simulink model "Position_Model"  (R2021a)
settings: Solver=VariableStepAuto  StartTime=0.0  StopTime=10.0  RelTol=1e-3
values from neighbouring files (symbols this model uses):
  Kr = 1.73    [TransferFunctionCode.m]    (also in run_steering_simulation.m)
  Kv = 0.53    [TransferFunctionCode.m]    (also in run_steering_simulation.m)
  phi_0 = 0    [run_steering_simulation.m]
  rhodot_d = 0.1    [run_steering_simulation.m]
  sigmar = 2.94    [TransferFunctionCode.m]    (also in run_steering_simulation.m)
  sigmav = 5.88    [TransferFunctionCode.m]    (also in run_steering_simulation.m)
  x_0 = 0    [run_steering_simulation.m]
  x_s = [0 3 6 10]    [run_steering_simulation.m]
  y_0 = 0    [run_steering_simulation.m]
  y_s = [0 0 3 3]    [run_steering_simulation.m]
libraries: pid_lib x3
settings Model: Creator=Brook Walls  LastModifiedBy=Brook Walls

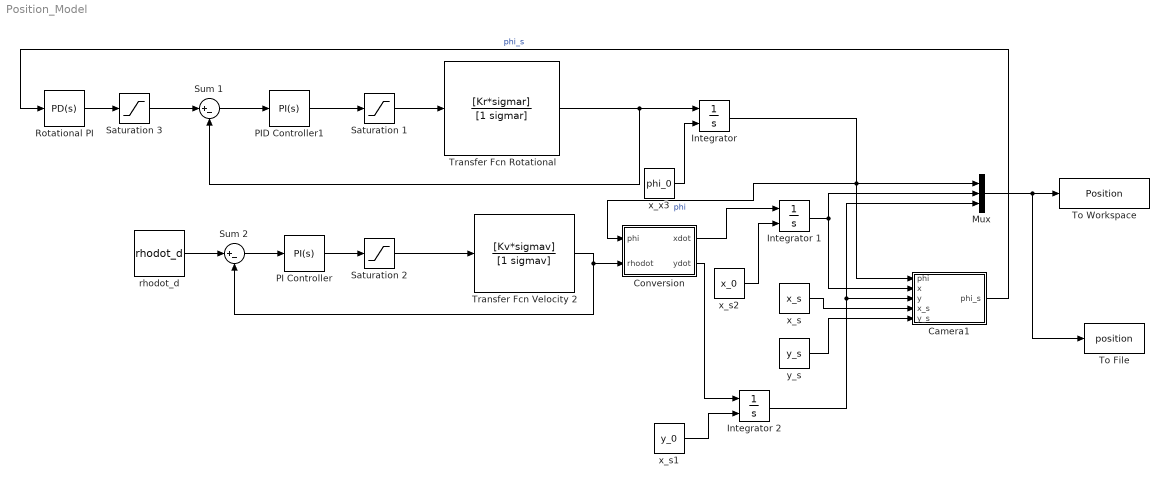
== system Position_Model ==
  Camera1 : MATLAB Function  TreatAsAtomicUnit=on  SystemSampleTime=.2
  Conversion : MATLAB Function  TreatAsAtomicUnit=on
  "Integrator " : Integrator  InitialConditionSource=external
  Integrator 1 : Integrator  InitialConditionSource=external
  Integrator 2 : Integrator  InitialConditionSource=external
  Mux : Mux  Inputs=3
  "PI Controller " : pid_lib/PID Controller  Controller=PI  Form=Parallel  TimeDomain=Continuous-time  UseExternalTs=off  SampleTime=-1  IntegratorMethod=Forward Euler  FilterMethod=Forward Euler  ControllerParametersSource=internal  P=3.69119211409962  I=0  D=0  UseFilter=on  N=100  TunerSelectOption=Transfer Function Based (PID Tuner App)  InitialConditionSource=internal  InitialConditionForIntegrator=0  InitialConditionForFilter=0  DifferentiatorICPrevScaledInput=0  ExternalReset=none  TrackingMode=off  Kt=1  LimitOutput=off  SatLimitsSource=internal  UpperSaturationLimit=inf  LowerSaturationLimit=-inf  LinearizeAsGain=on  AntiWindupMode=none  Kb=1  POutMin=[]  POutMax=[]  IOutMin=[]  IOutMax=[]  DOutMin=[]  DOutMax=[]  NOutMin=[]  NOutMax=[]  SumOutMin=[]  SumOutMax=[]  SaturationOutMin=[]  SaturationOutMax=[]  PParamMin=[]  PParamMax=[]  IParamMin=[]  IParamMax=[]  DParamMin=[]  DParamMax=[]  NParamMin=[]  NParamMax=[]  KbParamMin=[]  KbParamMax=[]  KtParamMin=[]  KtParamMax=[]  KbOutMin=[]  KbOutMax=[]  KtOutMin=[]  KtOutMax=[]  IntegratorOutMin=[]  IntegratorOutMax=[]  FilterOutMin=[]  FilterOutMax=[]  SumI1OutMin=[]  SumI1OutMax=[]  SumI2OutMin=[]  SumI2OutMax=[]  SumI3OutMin=[]  SumI3OutMax=[]  SumI4OutMin=[]  SumI4OutMax=[]  SumDOutMin=[]  SumDOutMax=[]  DifferentiatorOutMin=[]  DifferentiatorOutMax=[]  FilterDiffOutCoefMin=[]  FilterDiffOutCoefMax=[]  ReciprocalOutMin=[]  ReciprocalOutMax=[]  SumDenOutMin=[]  SumDenOutMax=[]  SumNumOutMin=[]  SumNumOutMax=[]  DivideOutMin=[]  DivideOutMax=[]  UdiffTsProdOutMin=[]  UdiffTsProdOutMax=[]  NTsProdOutMin=[]  NTsProdOutMax=[]  UintegralTsProdOutMin=[]  UintegralTsProdOutMax=[]  UngainTsProdOutMin=[]  UngainTsProdOutMax=[]  IntegratorContinuousStateAttributes=''  IntegratorStateMustResolveToSignalObject=off  IntegratorRTWStateStorageClass=Auto  FilterContinuousStateAttributes=''  FilterStateMustResolveToSignalObject=off  FilterRTWStateStorageClass=Auto  ParallelPVariant=InternalParameters  IdealPVariant=Disabled  IVariant=InternalParameters  DVariant=Disabled  IntegratorVariant=Continuous  SatVariant=Disabled  AWVariant=Passthrough  PCopyVariant=Disabled  TRVariant=Disabled  FdbkBlocksVariant=Forward  IdealPFdbkVariant=Disabled  SatFdbkVariant=Disabled  DerivativeFilterVariant=Disabled  NVariant=Disabled  NCopyVariant=Disabled_SignalSpec  FilterICVariant=Disabled  IntegratorICVariant=InternalICs  ExternalResetVariant=Disabled  TRSumVariant=Passthrough  SumFdbkVariant=Disabled  SumVariant=Sum_PI  TsampFilterVariant=InternalTs  TsampNgainVariant=Passthrough  TsampIntegralVariant=Passthrough  ExternalSaturationOutDataTypeStr=Inherit: Same as second input
  PID Controller1 : pid_lib/PID Controller  Controller=PI  Form=Parallel  TimeDomain=Continuous-time  UseExternalTs=off  SampleTime=-1  IntegratorMethod=Forward Euler  FilterMethod=Forward Euler  ControllerParametersSource=internal  P=2.17  I=0  D=0  UseFilter=on  N=100  TunerSelectOption=Transfer Function Based (PID Tuner App)  InitialConditionSource=internal  InitialConditionForIntegrator=0  InitialConditionForFilter=0  DifferentiatorICPrevScaledInput=0  ExternalReset=none  TrackingMode=off  Kt=1  LimitOutput=off  SatLimitsSource=internal  UpperSaturationLimit=inf  LowerSaturationLimit=-inf  LinearizeAsGain=on  AntiWindupMode=none  Kb=1  POutMin=[]  POutMax=[]  IOutMin=[]  IOutMax=[]  DOutMin=[]  DOutMax=[]  NOutMin=[]  NOutMax=[]  SumOutMin=[]  SumOutMax=[]  SaturationOutMin=[]  SaturationOutMax=[]  PParamMin=[]  PParamMax=[]  IParamMin=[]  IParamMax=[]  DParamMin=[]  DParamMax=[]  NParamMin=[]  NParamMax=[]  KbParamMin=[]  KbParamMax=[]  KtParamMin=[]  KtParamMax=[]  KbOutMin=[]  KbOutMax=[]  KtOutMin=[]  KtOutMax=[]  IntegratorOutMin=[]  IntegratorOutMax=[]  FilterOutMin=[]  FilterOutMax=[]  SumI1OutMin=[]  SumI1OutMax=[]  SumI2OutMin=[]  SumI2OutMax=[]  SumI3OutMin=[]  SumI3OutMax=[]  SumI4OutMin=[]  SumI4OutMax=[]  SumDOutMin=[]  SumDOutMax=[]  DifferentiatorOutMin=[]  DifferentiatorOutMax=[]  FilterDiffOutCoefMin=[]  FilterDiffOutCoefMax=[]  ReciprocalOutMin=[]  ReciprocalOutMax=[]  SumDenOutMin=[]  SumDenOutMax=[]  SumNumOutMin=[]  SumNumOutMax=[]  DivideOutMin=[]  DivideOutMax=[]  UdiffTsProdOutMin=[]  UdiffTsProdOutMax=[]  NTsProdOutMin=[]  NTsProdOutMax=[]  UintegralTsProdOutMin=[]  UintegralTsProdOutMax=[]  UngainTsProdOutMin=[]  UngainTsProdOutMax=[]  IntegratorContinuousStateAttributes=''  IntegratorStateMustResolveToSignalObject=off  IntegratorRTWStateStorageClass=Auto  FilterContinuousStateAttributes=''  FilterStateMustResolveToSignalObject=off  FilterRTWStateStorageClass=Auto  ParallelPVariant=InternalParameters  IdealPVariant=Disabled  IVariant=InternalParameters  DVariant=Disabled  IntegratorVariant=Continuous  SatVariant=Disabled  AWVariant=Passthrough  PCopyVariant=Disabled  TRVariant=Disabled  FdbkBlocksVariant=Forward  IdealPFdbkVariant=Disabled  SatFdbkVariant=Disabled  DerivativeFilterVariant=Disabled  NVariant=Disabled  NCopyVariant=Disabled_SignalSpec  FilterICVariant=Disabled  IntegratorICVariant=InternalICs  ExternalResetVariant=Disabled  TRSumVariant=Passthrough  SumFdbkVariant=Disabled  SumVariant=Sum_PI  TsampFilterVariant=InternalTs  TsampNgainVariant=Passthrough  TsampIntegralVariant=Passthrough  ExternalSaturationOutDataTypeStr=Inherit: Same as second input
  Rotational PI : pid_lib/PID Controller  Controller=PD  Form=Parallel  TimeDomain=Continuous-time  UseExternalTs=off  SampleTime=-1  IntegratorMethod=Forward Euler  FilterMethod=Forward Euler  ControllerParametersSource=internal  P=51.0923671487987  I=0  D=1.88750160017892  UseFilter=on  N=309.746780654974  TunerSelectOption=Transfer Function Based (PID Tuner App)  InitialConditionSource=internal  InitialConditionForIntegrator=0  InitialConditionForFilter=0  DifferentiatorICPrevScaledInput=0  ExternalReset=none  TrackingMode=off  Kt=1  LimitOutput=off  SatLimitsSource=internal  UpperSaturationLimit=inf  LowerSaturationLimit=-inf  LinearizeAsGain=on  AntiWindupMode=none  Kb=1  POutMin=[]  POutMax=[]  IOutMin=[]  IOutMax=[]  DOutMin=[]  DOutMax=[]  NOutMin=[]  NOutMax=[]  SumOutMin=[]  SumOutMax=[]  SaturationOutMin=[]  SaturationOutMax=[]  PParamMin=[]  PParamMax=[]  IParamMin=[]  IParamMax=[]  DParamMin=[]  DParamMax=[]  NParamMin=[]  NParamMax=[]  KbParamMin=[]  KbParamMax=[]  KtParamMin=[]  KtParamMax=[]  KbOutMin=[]  KbOutMax=[]  KtOutMin=[]  KtOutMax=[]  IntegratorOutMin=[]  IntegratorOutMax=[]  FilterOutMin=[]  FilterOutMax=[]  SumI1OutMin=[]  SumI1OutMax=[]  SumI2OutMin=[]  SumI2OutMax=[]  SumI3OutMin=[]  SumI3OutMax=[]  SumI4OutMin=[]  SumI4OutMax=[]  SumDOutMin=[]  SumDOutMax=[]  DifferentiatorOutMin=[]  DifferentiatorOutMax=[]  FilterDiffOutCoefMin=[]  FilterDiffOutCoefMax=[]  ReciprocalOutMin=[]  ReciprocalOutMax=[]  SumDenOutMin=[]  SumDenOutMax=[]  SumNumOutMin=[]  SumNumOutMax=[]  DivideOutMin=[]  DivideOutMax=[]  UdiffTsProdOutMin=[]  UdiffTsProdOutMax=[]  NTsProdOutMin=[]  NTsProdOutMax=[]  UintegralTsProdOutMin=[]  UintegralTsProdOutMax=[]  UngainTsProdOutMin=[]  UngainTsProdOutMax=[]  IntegratorContinuousStateAttributes=''  IntegratorStateMustResolveToSignalObject=off  IntegratorRTWStateStorageClass=Auto  FilterContinuousStateAttributes=''  FilterStateMustResolveToSignalObject=off  FilterRTWStateStorageClass=Auto  ParallelPVariant=InternalParameters  IdealPVariant=Disabled  IVariant=Disabled  DVariant=InternalParameters  IntegratorVariant=Disabled  SatVariant=Disabled  AWVariant=Disabled  PCopyVariant=Disabled  TRVariant=Disabled  FdbkBlocksVariant=Forward  IdealPFdbkVariant=Disabled  SatFdbkVariant=Disabled  DerivativeFilterVariant=ContFilter  NVariant=InternalParameters  NCopyVariant=Disabled  FilterICVariant=InternalICsFilter  IntegratorICVariant=Disabled  ExternalResetVariant=Disabled  TRSumVariant=Passthrough  SumFdbkVariant=Disabled  SumVariant=Sum_PD  TsampFilterVariant=InternalTs  TsampNgainVariant=Passthrough  TsampIntegralVariant=Disabled_SignalSpec  ExternalSaturationOutDataTypeStr=Inherit: Same as second input
  Saturation 1 : Saturate  UpperLimit=7.5  LowerLimit=-7.5
  Saturation 2 : Saturate  UpperLimit=7.5  LowerLimit=-7.5
  Saturation 3 : Saturate  UpperLimit=7.5  LowerLimit=-7.5
  Sum 1 : Sum  Inputs=|+-
  Sum 2 : Sum  Inputs=|+-
  "To File " : ToFile  Filename=position  MatrixName=velocity  SaveFormat=Timeseries  SampleTime=0
  To Workspace : ToWorkspace  VariableName=Position  SaveFormat=Timeseries  SampleTime=-1
  "Transfer Fcn Rotational " : TransferFcn  Numerator=[Kr*sigmar]  Denominator=[1 sigmar]
  Transfer Fcn Velocity 2 : TransferFcn  Numerator=[Kv*sigmav]  Denominator=[1 sigmav]
  rhodot_d : Constant  Value=rhodot_d
  x_s : Constant  Value=x_s
  x_s1 : Constant  Value=y_0
  x_s2 : Constant  Value=x_0
  x_x3 : Constant  Value=phi_0  VectorParams1D=off
  y_s : Constant  Value=y_s
  wires:
  Sum 2/1 -> "PI Controller "/1
  Sum 1/1 -> PID Controller1/1
  "Transfer Fcn Rotational "/1 -> Sum 1/2, "Integrator "/1
  x_x3/1 -> "Integrator "/2
  x_s2/1 -> Integrator 1/2
  Integrator 2/1 -> Camera1/3(y), Mux/3
  x_s1/1 -> Integrator 2/2
  Conversion/2(ydot) -> Integrator 2/1
  Conversion/1(xdot) -> Integrator 1/1
  Camera1/1(phi_s) -> Rotational PI/1  "phi_s"
  "Integrator "/1 -> Camera1/1(phi), Conversion/1(phi), Mux/1  "phi"
  Integrator 1/1 -> Camera1/2(x), Mux/2
  x_s/1 -> Camera1/4(x_s)
  Mux/1 -> "To File "/1, To Workspace/1
  rhodot_d/1 -> Sum 2/1
  Transfer Fcn Velocity 2/1 -> Sum 2/2, Conversion/2(rhodot)
  y_s/1 -> Camera1/5(y_s)
  PID Controller1/1 -> Saturation 1/1
  Saturation 1/1 -> "Transfer Fcn Rotational "/1
  "PI Controller "/1 -> Saturation 2/1
  Saturation 2/1 -> Transfer Fcn Velocity 2/1
  Saturation 3/1 -> Sum 1/1
  Rotational PI/1 -> Saturation 3/1

== matlab function Position_Model/Conversion ==
  data: xdot output; phi input; ydot output; rhodot input
function [xdot, ydot]= fcn(phi, rhodot)

xdot = rhodot*cos(phi*pi/180);
ydot = rhodot*sin(phi*pi/180);

y = phi;

== matlab function Position_Model/Camera1 ==
  data: phi input; phi_s output; x input; y input; x_s input; y_s input
function phi_s = fcn(phi,x,y,x_s,y_s)
%#codegen
%
% Simulation of Camera with line detection
% phi - angle of robot in degrees
% x - x position of robot in feet
% y - y position of robot in feet
% x_s - vector of x coordinates for line to be detected (in feet)
% y_s - vector of y coordinates for line to be detected (in feet)
%
%

% change show_image to 1 to see camera image during simulation
show_image=1;
%
% number of horizontal and vertical pixels
%
h_pix = 740;
v_pix = 480;
%
% pixel_check is the row of the image to check for the line (origin of
% camera image is upper right
% 
pixel_check = v_pix*4/5;
%
% meters to feet conversion
%
mtof = 3.28;
% f is focal length 
%
f = .0036; %m
f = mtof*f; % convert to feet
%
% sensor image area
%
image_w = .00376; % m
image_h = .00274; % m
image_w = image_w*mtof; % convert to feet
image_h = image_h*mtof; % convert to feet
%
% h is height of the camera 
%
h = 0.1; % m
h = h*mtof; % convert to feet
%
% angle of view is from center to edge of camrea in radians
%
angle_of_view=53.5; % degrees

%
% interpolate between line points
%
x_s = interp1q((1:length(x_s))',x_s,(1:.01:length(x_s))');
y_s = interp1q((1:length(y_s))',y_s,(1:.01:length(y_s))');
%
% translate points to camera origin
% 
tape=[x_s,y_s]';
% figure
% plot(tape(1,:),tape(2,:),'*')
% axis([-5 5 -5 5])

tape = tape - [x;y]*ones(1,size(tape,2));
% figure
% plot(tape(1,:),tape(2,:),'*')
% axis([-5 5 -5 5])
%
% find points that are in the angle of view
%
angle = (180/pi)*acos(([cos(phi*pi/180) sin(phi*pi/180)]*tape)./sqrt(sum(tape.^2)));
index=find(angle<angle_of_view/2 & angle>-angle_of_view/2);
if isempty(index)
    disp('Tape not visible to the robot')
    phi_s = 0;
    return
end;
tape=tape(:,index);
% figure
% plot(tape(1,:),tape(2,:),'*')
% hold on
% fill(v_c(1,:),v_c(2,:),'y')
% title('visible points')
% axis([-5 5 -5 5])
%
% rotate points so straight ahead is along x axis
%
tapenorm=[cos(phi*pi/180) sin(phi*pi/180);-sin(phi*pi/180) cos(phi*pi/180)]*tape;
%
% map onto film coordinates
%
image = [(f./tapenorm(1,:)).*(-tapenorm(2,:));
    (f./tapenorm(1,:)).*(-h*ones(1,size(tapenorm,2)))];
% figure
% plot(image(1,:),image(2,:),'*')
% axis([-image_w/2 image_w/2 -image_h/2 image_h/2])

%
% map onto pixel coordinates
%
pixel = [0; v_pix]*ones(1,size(image,2)) + diag([h_pix/image_w -v_pix/image_h])*image+[h_pix/2; -v_pix/2]*ones(1,size(image,2));
if (show_image)
 figure(1)
 plot(pixel(1,:),pixel(2,:),'*')
 set(gca, 'YDir','reverse')
 hold on
 plot([0 h_pix],[pixel_check pixel_check],'r-')
 axis([0 h_pix 0 v_pix])
 hold off
 title('Robot camera view set show_image=0 to turn off and speed up simulation','interpreter','none')
end;


%
% find point on horizontal line at pixel number pixel_check
%
checkpoints= find(pixel(2,:)>=pixel_check);
if ~isempty(checkpoints)
    [m,index]=min(pixel(2,checkpoints));  
    if abs(pixel(2,index)-pixel_check)>10,
        disp(['no point visible near row ',int2str(pixel_check)])
        phi_s = 0;
        return
    end;
else
    disp(['no point visible near row ',int2str(pixel_check)])
    phi_s = 0;
    return
end;


phi_s = -(pixel(1,index)-h_pix/2)*angle_of_view/h_pix;
